simulink model "Tracker_old_version"  (R2021b)
settings: Solver=VariableStepAuto  StartTime=0.0  StopTime=10.0  RelTol=1e-3
libraries: raspberrypiNetworklib x2, realtime_pacer_lib x1
settings Model: Creator=Blade  LastModifiedBy=Blade

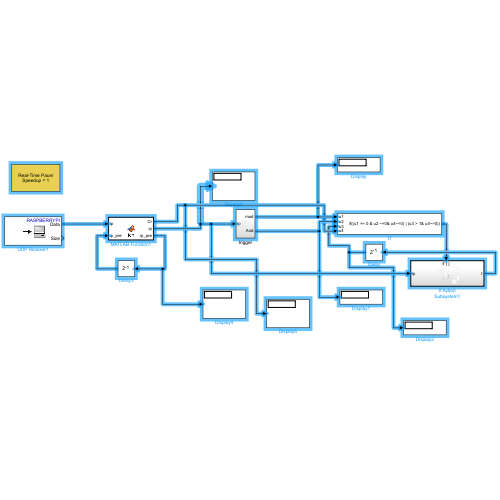
[thumbnail: Simulink's stored preview of the top-level diagram]
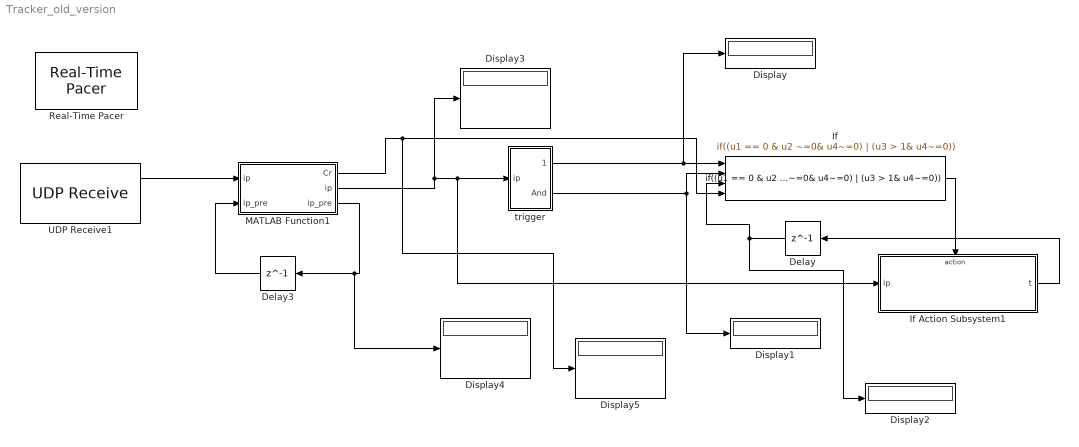
== system Tracker_old_version ==
  Delay : Delay  DelayLength=1  InitialCondition=0
  Delay3 : Delay  DelayLength=1  InitialCondition=0
  Display{,1..5} (6 alike) : Display
  If : If  NumInputs=4  IfExpression=(u1 == 0 & u2 ~=0& u4~=0) | (u3 > 1& u4~=0)  ShowElse=off
  If Action Subsystem1 : Subsystem  TreatAsAtomicUnit=on
  MATLAB Function1 : MATLAB Function  TreatAsAtomicUnit=on
  Real-Time Pacer : realtime_pacer_lib/Real-Time Pacer  simTimePerRealTime=1
      settings: SourceProductName=Real-Time Pacer
  UDP Receive1 : raspberrypiNetworklib/UDP Receive  localURL='0.0.0.0'  localPort=1000  remoteURL='0.0.0.0'  remotePort=-1  recvBufferSize=8192  signalDatatype=double  dims=2  isVarSize=off  showBlockingTime=off  blockingTime=0  sampletime=-1  blockPlatform=Raspberry Pi
      settings: SourceProductBaseCode=RASPPI
  trigger : Subsystem
  wires:
  If Action Subsystem1/1(t) -> Delay/1
  MATLAB Function1/1(Cr) -> Display5/1, If/4
  MATLAB Function1/3(ip_pre) -> Display4/1, Delay3/1
  trigger/1(mod) -> If/1, Display/1
  UDP Receive1/1 -> MATLAB Function1/1("ip ")
  If/1 -> If Action Subsystem1/Action
  trigger/2(And) -> If/2, Display1/1
  Delay/1 -> Display2/1, If/3
  Delay3/1 -> MATLAB Function1/2("ip_pre ")
  MATLAB Function1/2(ip) -> Display3/1, If Action Subsystem1/1(ip), trigger/1(ip)

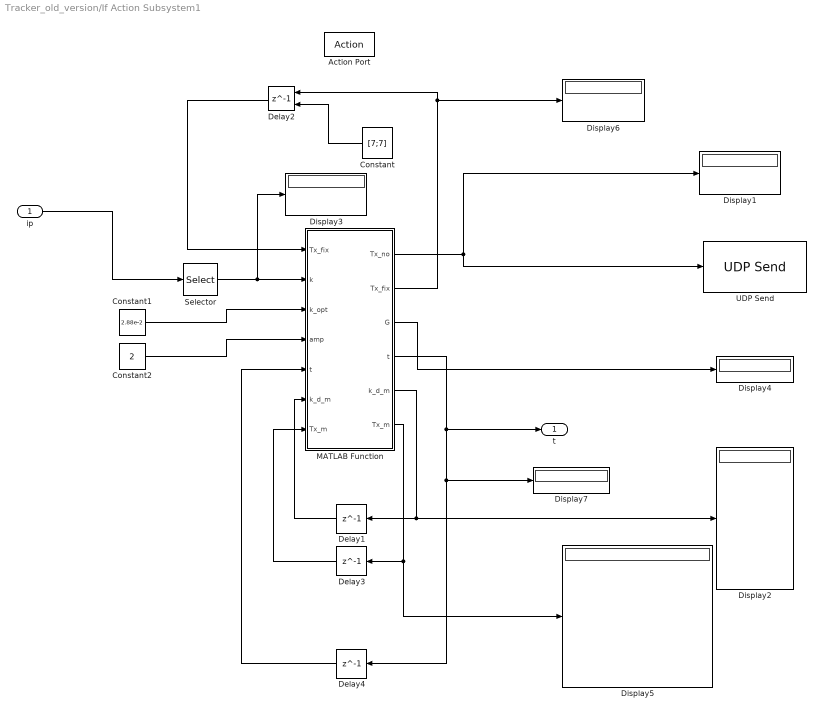
== system Tracker_old_version/If Action Subsystem1 ==
  ip : Inport
  Action Port : ActionPort  ActionPortLabel=if((u1 == 0 & u2 ~=0& u4~=0) | (u3 > 1& u4~=0))
  Constant : Constant  Value=[7;7]  VectorParams1D=off
  Constant1 : Constant  Value=2.88e-2
  Constant2 : Constant  Value=2
  Delay1 : Delay  DelayLength=1  InitialCondition=zeros(1,9)
  Delay2 : Delay  DelayLength=1  InitialConditionSource=Input port  InitialCondition=0
      settings: InputPortMap=u0,p4
  Delay3 : Delay  DelayLength=1  InitialCondition=zeros(8,2)
  Delay4 : Delay  DelayLength=1  InitialCondition=0
  Display{1..7} (7 alike) : Display
  MATLAB Function : MATLAB Function  TreatAsAtomicUnit=on
  Selector : Selector  InputPortWidth=2  IndexOptions=Index vector (dialog)  Indices=1  OutputSizes=1
  UDP Send : raspberrypiNetworklib/UDP Send  remoteURL='172.20.10.2'  remotePort=2000  localURL='0.0.0.0'  localPortSource=Automatically determine  localPort=-1  sampletime=-1  blockPlatform=Raspberry Pi  separateLengthPort=0
      settings: SourceProductBaseCode=RASPPI
  t : Outport
  wires:
  Delay4/1 -> MATLAB Function/5("t ")
  Constant2/1 -> MATLAB Function/4(amp)
  ip/1 -> Selector/1
  Constant1/1 -> MATLAB Function/3(k_opt)
  Delay2/1 -> MATLAB Function/1("Tx_fix ")
  MATLAB Function/1(Tx_no) -> UDP Send/1, Display1/1
  MATLAB Function/4(t) -> Display7/1, Delay4/1, t/1
  MATLAB Function/5(k_d_m) -> Delay1/1, Display2/1
  MATLAB Function/6(Tx_m) -> Display5/1, Delay3/1
  Selector/1 -> Display3/1, MATLAB Function/2(k)
  Delay1/1 -> MATLAB Function/6("k_d_m ")
  MATLAB Function/2(Tx_fix) -> Display6/1, Delay2/1
  Constant/1 -> Delay2/2
  MATLAB Function/3(G) -> Display4/1
  Delay3/1 -> MATLAB Function/7("Tx_m ")

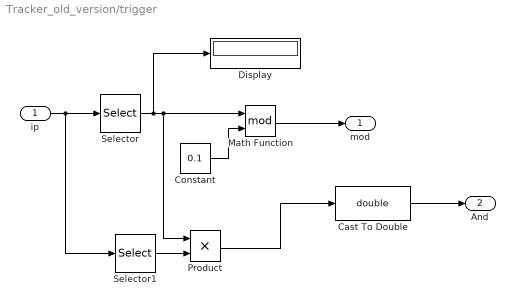
== system Tracker_old_version/trigger ==
  ip : Inport
  Cast To Double : DataTypeConversion  OutDataTypeStr=double
  Constant : Constant  Value=0.1
  Display : Display
  Math Function : Math  Operator=mod  SaturateOnIntegerOverflow=on
  Product : Product
  Selector : Selector  InputPortWidth=2  IndexOptions=Index vector (dialog)  Indices=2  OutputSizes=1
  Selector1 : Selector  InputPortWidth=2  IndexOptions=Index vector (dialog)  Indices=1  OutputSizes=1
  mod : Outport
  And : Outport  Port=2
  wires:
  Constant/1 -> Math Function/2
  Selector/1 -> Display/1, Product/1, Math Function/1
  ip/1 -> Selector1/1, Selector/1
  Math Function/1 -> mod/1
  Product/1 -> Cast To Double/1
  Selector1/1 -> Product/2
  Cast To Double/1 -> And/1

== matlab function Tracker_old_version/MATLAB Function1 ==
  data: Cr output; ip output; ip input; ip_pre input; ip_pre output
function [Cr,ip, ip_pre] = fcn(ip, ip_pre)

ip2 = ip(2);

if ip2 == ip_pre
    Cr = 0;
else
    ip_pre = ip2;
    Cr = 1;

end

== matlab function Tracker_old_version/If Action Subsystem1/MATLAB Function ==
  data: Tx_fix input; k input; Tx_no output; Tx_fix output; G output; t output; k_opt input; amp input; t input; k_d_m output; k_d_m input; Tx_m input; Tx_m output
function [Tx_no,Tx_fix,G,t,k_d_m,Tx_m] = Controller(Tx_fix,k,k_opt,amp,t,k_d_m,Tx_m)

k_diff = abs(k_opt-k)/k_opt;
G = round(amp*k_d_m(1));

if t ~=0
    
    k_d_m (t-1) = k_diff;
  
else

    t = t+1;

end


if t < 10
    if t < 9

        dir_att = [-1,-1; -1,0; 0,-1; 1,1; 1,0; 0,1; 1,-1; -1,1];
        
        
        Tx_no =G*dir_att(t,:)'+Tx_fix;
    
        Tx_m (t,:) = Tx_no;
    else
         Tx_no = Tx_fix;

    end
    t =t+1;

else
    
    dir_cand = [0,0; -1,-1; -1,0; 0,-1; 1,1; 1,0; 0,1; 1,-1; -1,1]; 
    [~, index] = min(k_d_m);
    dir_opt = dir_cand(index,:);
    G = round(amp*k_d_m(1));
    Tx_no = Tx_fix+ dir_opt'*G;
    Tx_fix = Tx_no;
    t =0;
   
 
end
